simulink model "trayectoria_desde_Velocidades"  (R2022a)
settings: Solver=VariableStepAuto  StartTime=0.0  StopTime=1739  RelTol=1e-3
values from neighbouring files (symbols this model uses):
  fs = 1/3    (= 0.333333333333)    [p2.m]
settings Model: Creator=jorch  LastModifiedBy=jorch

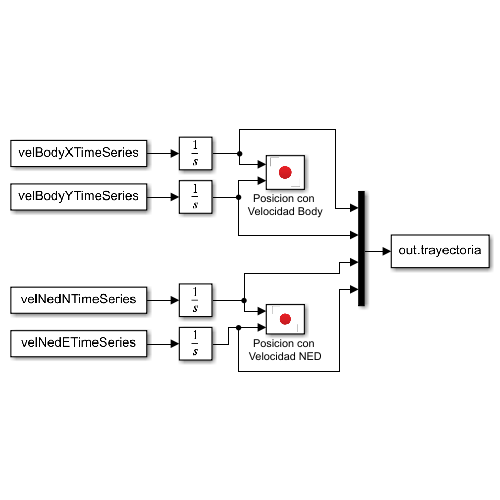
[thumbnail: Simulink's stored preview of the top-level diagram]
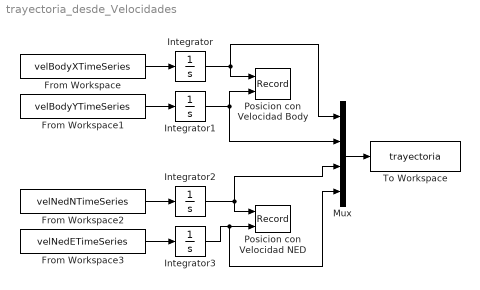
== system trayectoria_desde_Velocidades ==
  From Workspace : FromWorkspace  VariableName=velBodyXTimeSeries  SampleTime=fs
  From Workspace1 : FromWorkspace  VariableName=velBodyYTimeSeries  SampleTime=fs
  From Workspace2 : FromWorkspace  VariableName=velNedNTimeSeries  SampleTime=fs
  From Workspace3 : FromWorkspace  VariableName=velNedETimeSeries  SampleTime=fs
  Integrator{,1..3} (4 alike) : Integrator
  Mux : Mux
  Posicion con Velocidad Body : Record  FileSettingsInternal="{\"entries\":[{\"content\":{\"excelSettings\":{\"content\":{},\"type\":\"Streamout.ExcelSettings\"}},\"type\":\"Streamout.FileSettingStorage\",\"uuid\":\"828a547a-7f60-43d8-b5a3-15e1f5150f29\"}],\"packageUris\":[\"http://schema.mathworks.com/mf0/streamout_blocks/R2020a\"],\"version\":\"1.0\"}"  Layout=[1 1]  SignalsInternal="{\"entries\":[{\"content\":{\"signals\":[{\"content\":{\"blockPath\":[\"untitled/XY Graph\"],\"channel\":[],\"dimensions\":[1],\"domain\":\"untitled/XY Graph\",\"lineColor\":\"#a2142f\",\"plots\":[1],\"port\":1,\"sid\":[\"\"],\"signalID\":36,\"signalName\":\"Integrator\"},\"type\":\"RecordBlkView.Signal\",\"uuid\":\"8dc54bb3-0d88-44fc-a93f-1ad2288210e1\"},{\"content\":{\"blockPath\":[\"untitled/XY Graph\"],\"channel\":[],\"dimensions\":[1],\"domain\":\"untitled/XY Graph\",\"lineColor\":\"#139fff\",\"plots\":[1],\"port\":2,\"sid\":[\"\"],\"signalID\":40,\"signalName\":\"Integrator1\"},\"type\":\"RecordBlkView.Signal\",\"uuid\":\"34e5b253-150c-4d5f-a66d-d58e83e2e310\"}]},\"type\":\"RecordBlkView.InputSignals\",\"uuid\":\"aebbd936-5f30-4931-b675-127c6236c04f\"}],\"packageUris\":[\"http://schema.mathworks.com/mf0/streamout_blocks/R2020a\"],\"version\":\"1.0\"}"  VisualizationBindings="{\"xyplotplugin\":{\"info\":[{\"series\":[{\"bindingParametersList\":[{\"parameter\":\"X-Axis\",\"signalID\":36,\"signalName\":\"Integrator\"},{\"parameter\":\"Y-Axis\",\"signalID\":40,\"signalName\":\"Integrator1\"}],\"seriesID\":2415}],\"subplotID\":1}]}}"  CompatibilityTag=XY
  Posicion con Velocidad NED : Record  FileSettingsInternal="{\"entries\":[{\"content\":{\"excelSettings\":{\"content\":{},\"type\":\"Streamout.ExcelSettings\"}},\"type\":\"Streamout.FileSettingStorage\",\"uuid\":\"b55d006b-e9c0-4ac5-86c3-c46564886c33\"}],\"packageUris\":[\"http://schema.mathworks.com/mf0/streamout_blocks/R2020a\"],\"version\":\"1.0\"}"  Layout=[1 1]  SignalsInternal="{\"entries\":[{\"content\":{\"signals\":[{\"content\":{\"blockPath\":[\"untitled/XY Graph1\"],\"channel\":[],\"dimensions\":[1],\"domain\":\"untitled/XY Graph1\",\"lineColor\":\"#a2142f\",\"plots\":[1],\"port\":1,\"sid\":[\"\"],\"signalID\":44,\"signalName\":\"Integrator2\"},\"type\":\"RecordBlkView.Signal\",\"uuid\":\"54edf679-09b6-4382-8954-5681d495bfd1\"},{\"content\":{\"blockPath\":[\"untitled/XY Graph1\"],\"channel\":[],\"dimensions\":[1],\"domain\":\"untitled/XY Graph1\",\"lineColor\":\"#139fff\",\"plots\":[1],\"port\":2,\"sid\":[\"\"],\"signalID\":48,\"signalName\":\"Integrator3\"},\"type\":\"RecordBlkView.Signal\",\"uuid\":\"95ad90bf-5b1b-4eb9-938c-d61d2ece4182\"}]},\"type\":\"RecordBlkView.InputSignals\",\"uuid\":\"e446679c-adff-47b7-a5f4-e1078dcda577\"}],\"packageUris\":[\"http://schema.mathworks.com/mf0/streamout_blocks/R2020a\"],\"version\":\"1.0\"}"  VisualizationBindings="{\"xyplotplugin\":{\"info\":[{\"series\":[{\"bindingParametersList\":[{\"parameter\":\"X-Axis\",\"signalID\":44,\"signalName\":\"Integrator2\"},{\"parameter\":\"Y-Axis\",\"signalID\":48,\"signalName\":\"Integrator3\"}],\"seriesID\":24499}],\"subplotID\":1}]}}"  CompatibilityTag=XY
  To Workspace : ToWorkspace  VariableName=trayectoria  SampleTime=fs
  wires:
  From Workspace/1 -> Integrator/1
  From Workspace1/1 -> Integrator1/1
  From Workspace2/1 -> Integrator2/1
  From Workspace3/1 -> Integrator3/1
  Integrator/1 -> Mux/1, Posicion con Velocidad Body/1
  Integrator1/1 -> Mux/2, Posicion con Velocidad Body/2
  Integrator2/1 -> Posicion con Velocidad NED/1, Mux/3
  Integrator3/1 -> Mux/4, Posicion con Velocidad NED/2
  Mux/1 -> To Workspace/1
